simulink model "TorqueVectoring_6_1"  (R2023a)
settings: Solver=FixedStepAuto  StartTime=0.0  StopTime=8  FixedStep=.001  RelTol=1e-3
model workspace (MAT data in the model file):
  slipTarget : Simulink.Parameter (value not decoded)
values from neighbouring files (symbols this model uses):
  Kd_slip = 0    [Main_TorqueVectoring_5_1.m]
  Kd_yaw = 0    [Main_TorqueVectoring_5_1.m]
  Ki_slip = 50    [Main_TorqueVectoring_5_1.m]
  Ki_yaw = 10    [Main_TorqueVectoring_5_1.m]
  Kp_slip = 250    [Main_TorqueVectoring_5_1.m]
  Kp_yaw = 100    [Main_TorqueVectoring_5_1.m]
  slip_windupLower = -inf    [Main_TorqueVectoring_5_1.m]
  slip_windupUpper = inf    [Main_TorqueVectoring_5_1.m]
  slipTarget = .2    (= 0.2)    [Main_TorqueVectoring_5_1.m]
  steering = table2array(yawrateSteering)    [Main_TorqueVectoring_5_1.m]
  yaw_prev_error = 0    [Main_TorqueVectoring_5_1.m]
  yawRate = table2array(yawrateTable)    [Main_TorqueVectoring_5_1.m]
  yawrateVelocity = [0, 5, 10, 15, 20, 25, 30, 35]    [Main_TorqueVectoring_5_1.m]
undefined symbols (not defined in the file or in its folder): sigbuilder_block, VehicleVelocity
libraries: slpidlib x6
(part 3 of 4)

== system TorqueVectoring_6_1/Vehicle Dynamics Model/14 DOF MODEL/Subsys Tire/Subsys tfl2/Subsys Fx ==
  note: B
  note: Bx
  note: Bx - atanBX
  note: X
  note: x
  S : Inport
  Fz : Inport  Port=2
  Bx : Product  RndMeth=Zero
  C : Constant  Value=1.65
  Divide : Product  Inputs=*/
  Gain : Gain  Gain=100
  Product{1..4} (4 alike) : Product  RndMeth=Zero
  Scope2 : Scope
  Sh2 : Constant  Value=0
  Subsys BCD : Subsystem
  Subsys D : Subsystem
  SubsysE : Subsystem
  Subtract : Sum  Inputs=+-
  Subtract1 : Sum  Inputs=+-
  Subtract3 : Sum
  Subtract4 : Sum
  Sv : Constant  Value=0
  To Workspace1 : ToWorkspace  VariableName=Fxrls  SampleTime=-1
  atan : Trigonometry  Operator=atan
  atanBx : Trigonometry  Operator=atan
  atanBx1 : Trigonometry
  Fx : Outport
  wires:
  C/1 -> Product2/1, Product3/2
  Subsys D/1(D) -> Product2/2, Product4/2
  Subsys BCD/1(BCD) -> Divide/1
  Product2/1 -> Divide/2
  Subtract3/1 -> Scope2/1, To Workspace1/1, Fx/1
  Product4/1 -> Subtract3/1
  Product3/1 -> atanBx1/1
  atanBx1/1 -> Product4/1
  atan/1 -> Product3/1
  S/1 -> Gain/1
  Subtract4/1 -> Bx/1
  Sv/1 -> Subtract3/2
  Subtract1/1 -> atan/1
  Product1/1 -> Subtract1/2
  SubsysE/1(E) -> Product1/2
  Subtract/1 -> Product1/1
  atanBx/1 -> Subtract/2
  Bx/1 -> Subtract/1, Subtract1/1, atanBx/1
  Divide/1 -> Bx/2
  Sh2/1 -> Subtract4/2
  Fz/1 -> Subsys BCD/1(Fz), Subsys D/1(Fz), SubsysE/1(Fz)
  Gain/1 -> Subtract4/1

== system TorqueVectoring_6_1/Vehicle Dynamics Model/14 DOF MODEL/Subsys Tire/Subsys tfl2/Subsys Fy ==
  note: B
  note: Bx
  note: Bx - atanBX
  note: X
  note: x
  note: Sh
  alpha : Inport
  Fz : Inport  Port=2
  Bx : Product  RndMeth=Zero
  C : Constant  Value=1.3
  Divide : Product  Inputs=*/
  Product{1..4} (4 alike) : Product  RndMeth=Zero
  Scope2 : Scope
  Subsys BCD : Subsystem
  Subsys D : Subsystem
  SubsysE : Subsystem
  Subtract : Sum  Inputs=+-
  Subtract1 : Sum  Inputs=+-
  Subtract3 : Sum
  Subtract4 : Sum
  Sv : Constant  Value=0
  Sv1 : Constant  Value=0
  To Workspace1 : ToWorkspace  VariableName=Fyrls  SampleTime=-1
  atan : Trigonometry  Operator=atan
  atanBx : Trigonometry  Operator=atan
  atanBx1 : Trigonometry
  Fy : Outport
  wires:
  C/1 -> Product2/1, Product3/2
  Subsys D/1(D) -> Product2/2, Product4/2
  Product2/1 -> Divide/2
  Subtract3/1 -> Scope2/1, To Workspace1/1, Fy/1
  Product4/1 -> Subtract3/1
  Product3/1 -> atanBx1/1
  atanBx1/1 -> Product4/1
  atan/1 -> Product3/1
  Subtract4/1 -> Bx/1
  Sv/1 -> Subtract3/2
  Subtract1/1 -> atan/1
  Product1/1 -> Subtract1/2
  SubsysE/1(E) -> Product1/2
  Subtract/1 -> Product1/1
  atanBx/1 -> Subtract/2
  Bx/1 -> Subtract/1, Subtract1/1, atanBx/1
  Divide/1 -> Bx/2
  Sv1/1 -> Subtract4/2
  Subsys BCD/1(BCD) -> Divide/1
  alpha/1 -> Subtract4/1
  Fz/1 -> Subsys BCD/1(Fz), Subsys D/1(Fz), SubsysE/1(Fz)

== system TorqueVectoring_6_1/Vehicle Dynamics Model/14 DOF MODEL/Subsys Tire/Subsys tfl2/Subsys Mz ==
  note: B
  note: Bx
  note: Bx - atanBX
  note: X
  note: x
  alpha : Inport
  Fz : Inport  Port=2
  Bx : Product  RndMeth=Zero
  C : Constant  Value=2.40
  Divide : Product  Inputs=*/
  Product{1..4} (4 alike) : Product  RndMeth=Zero
  Scope2 : Scope
  Sh2 : Constant  Value=0
  Subsys BCD : Subsystem
  Subsys D : Subsystem
  SubsysE : Subsystem
  Subtract : Sum  Inputs=+-
  Subtract1 : Sum  Inputs=+-
  Subtract3 : Sum
  Subtract4 : Sum
  Sv2 : Constant  Value=0
  To Workspace1 : ToWorkspace  VariableName=Mzrls  SampleTime=-1
  atan : Trigonometry  Operator=atan
  atanBx : Trigonometry  Operator=atan
  atanBx1 : Trigonometry
  Mz : Outport
  wires:
  C/1 -> Product2/1, Product3/2
  Subsys D/1(D) -> Product2/2, Product4/2
  Subsys BCD/1(BCD) -> Divide/1
  Product2/1 -> Divide/2
  Subtract3/1 -> Scope2/1, To Workspace1/1, Mz/1
  Product4/1 -> Subtract3/1
  Product3/1 -> atanBx1/1
  atanBx1/1 -> Product4/1
  atan/1 -> Product3/1
  alpha/1 -> Subtract4/1
  Subtract4/1 -> Bx/1
  Sv2/1 -> Subtract3/2
  Subtract1/1 -> atan/1
  Product1/1 -> Subtract1/2
  SubsysE/1(E) -> Product1/2
  Subtract/1 -> Product1/1
  atanBx/1 -> Subtract/2
  Bx/1 -> Subtract/1, Subtract1/1, atanBx/1
  Divide/1 -> Bx/2
  Sh2/1 -> Subtract4/2
  Fz/1 -> Subsys BCD/1(Fz), Subsys D/1(Fz), SubsysE/1(Fz)

== system TorqueVectoring_6_1/Vehicle Dynamics Model/14 DOF MODEL/Subsys Tire/Subsys tfl3/Subsys Fx ==
  note: x
  note: X
  note: Bx - atanBX
  note: Bx
  note: B
  S : Inport
  Fz : Inport  Port=2
  Bx : Product  RndMeth=Zero
  C : Constant  Value=1.65
  Divide : Product  Inputs=*/
  Gain : Gain  Gain=100
  Product{1..4} (4 alike) : Product  RndMeth=Zero
  Scope2 : Scope
  Sh2 : Constant  Value=0
  Subsys BCD : Subsystem
  Subsys D : Subsystem
  SubsysE : Subsystem
  Subtract : Sum  Inputs=+-
  Subtract1 : Sum  Inputs=+-
  Subtract3 : Sum
  Subtract4 : Sum
  Sv : Constant  Value=0
  To Workspace1 : ToWorkspace  VariableName=Fxrrs  SampleTime=-1
  atan : Trigonometry  Operator=atan
  atanBx : Trigonometry  Operator=atan
  atanBx1 : Trigonometry
  Fx : Outport
  wires:
  Gain/1 -> Subtract4/1
  Fz/1 -> SubsysE/1(Fz), Subsys D/1(Fz), Subsys BCD/1(Fz)
  Sh2/1 -> Subtract4/2
  Divide/1 -> Bx/2
  Bx/1 -> atanBx/1, Subtract1/1, Subtract/1
  atanBx/1 -> Subtract/2
  Subtract/1 -> Product1/1
  SubsysE/1(E) -> Product1/2
  Product1/1 -> Subtract1/2
  Subtract1/1 -> atan/1
  Sv/1 -> Subtract3/2
  Subtract4/1 -> Bx/1
  S/1 -> Gain/1
  atan/1 -> Product3/1
  atanBx1/1 -> Product4/1
  Product3/1 -> atanBx1/1
  Product4/1 -> Subtract3/1
  Subtract3/1 -> To Workspace1/1, Fx/1, Scope2/1
  Product2/1 -> Divide/2
  Subsys BCD/1(BCD) -> Divide/1
  Subsys D/1(D) -> Product4/2, Product2/2
  C/1 -> Product3/2, Product2/1

== system TorqueVectoring_6_1/Vehicle Dynamics Model/14 DOF MODEL/Subsys Tire/Subsys tfl3/Subsys Fy ==
  note: Sh
  note: x
  note: X
  note: Bx - atanBX
  note: Bx
  note: B
  alpha : Inport
  Fz : Inport  Port=2
  Bx : Product  RndMeth=Zero
  C : Constant  Value=1.3
  Divide : Product  Inputs=*/
  Product{1..4} (4 alike) : Product  RndMeth=Zero
  Scope2 : Scope
  Subsys BCD : Subsystem
  Subsys D : Subsystem
  SubsysE : Subsystem
  Subtract : Sum  Inputs=+-
  Subtract1 : Sum  Inputs=+-
  Subtract3 : Sum
  Subtract4 : Sum
  Sv : Constant  Value=0
  Sv1 : Constant  Value=0
  To Workspace1 : ToWorkspace  VariableName=Fyrrs  SampleTime=-1
  atan : Trigonometry  Operator=atan
  atanBx : Trigonometry  Operator=atan
  atanBx1 : Trigonometry
  Fy : Outport
  wires:
  Fz/1 -> SubsysE/1(Fz), Subsys D/1(Fz), Subsys BCD/1(Fz)
  alpha/1 -> Subtract4/1
  Subsys BCD/1(BCD) -> Divide/1
  Sv1/1 -> Subtract4/2
  Divide/1 -> Bx/2
  Bx/1 -> atanBx/1, Subtract1/1, Subtract/1
  atanBx/1 -> Subtract/2
  Subtract/1 -> Product1/1
  SubsysE/1(E) -> Product1/2
  Product1/1 -> Subtract1/2
  Subtract1/1 -> atan/1
  Sv/1 -> Subtract3/2
  Subtract4/1 -> Bx/1
  atan/1 -> Product3/1
  atanBx1/1 -> Product4/1
  Product3/1 -> atanBx1/1
  Product4/1 -> Subtract3/1
  Subtract3/1 -> Fy/1, To Workspace1/1, Scope2/1
  Product2/1 -> Divide/2
  Subsys D/1(D) -> Product4/2, Product2/2
  C/1 -> Product3/2, Product2/1

== system TorqueVectoring_6_1/Vehicle Dynamics Model/14 DOF MODEL/Subsys Tire/Subsys tfl3/Subsys Mz ==
  note: x
  note: X
  note: Bx - atanBX
  note: Bx
  note: B
  alpha : Inport
  Fz : Inport  Port=2
  Bx : Product  RndMeth=Zero
  C : Constant  Value=2.40
  Divide : Product  Inputs=*/
  Product{1..4} (4 alike) : Product  RndMeth=Zero
  Scope2 : Scope
  Sh2 : Constant  Value=0
  Subsys BCD : Subsystem
  Subsys D : Subsystem
  SubsysE : Subsystem
  Subtract : Sum  Inputs=+-
  Subtract1 : Sum  Inputs=+-
  Subtract3 : Sum
  Subtract4 : Sum
  Sv2 : Constant  Value=0
  To Workspace1 : ToWorkspace  VariableName=Mzrrs  SampleTime=-1
  atan : Trigonometry  Operator=atan
  atanBx : Trigonometry  Operator=atan
  atanBx1 : Trigonometry
  Mz : Outport
  wires:
  Fz/1 -> SubsysE/1(Fz), Subsys D/1(Fz), Subsys BCD/1(Fz)
  Sh2/1 -> Subtract4/2
  Divide/1 -> Bx/2
  Bx/1 -> atanBx/1, Subtract1/1, Subtract/1
  atanBx/1 -> Subtract/2
  Subtract/1 -> Product1/1
  SubsysE/1(E) -> Product1/2
  Product1/1 -> Subtract1/2
  Subtract1/1 -> atan/1
  Sv2/1 -> Subtract3/2
  Subtract4/1 -> Bx/1
  alpha/1 -> Subtract4/1
  atan/1 -> Product3/1
  atanBx1/1 -> Product4/1
  Product3/1 -> atanBx1/1
  Product4/1 -> Subtract3/1
  Subtract3/1 -> Mz/1, To Workspace1/1, Scope2/1
  Product2/1 -> Divide/2
  Subsys BCD/1(BCD) -> Divide/1
  Subsys D/1(D) -> Product4/2, Product2/2
  C/1 -> Product3/2, Product2/1

== system TorqueVectoring_6_1/Vehicle Dynamics Model/14 DOF MODEL/Subsys ride/Subsys Fz/Subsys Fzfl ==
  note: mufl.g
  note: Ms.g
  note: Ms.gb
  note: a+b
  note: 2(a+b)
  note: Msg.b/2(a+b)
  Ffl : Inport
  Add : Sum
  Add1 : Sum  Inputs=+++
  Divide : Product  Inputs=*/
  Ms : Constant  Value=Ms
  Product3 : Product  RndMeth=Zero
  a : Constant  Value=a
  b : Constant  Value=b
  constant : Gain  Gain=2
  g : Gain  Gain=9.81
  g1 : Gain  Gain=9.81
  mufl : Constant  Value=mufl
  Fzfl : Outport
  wires:
  b/1 -> Product3/2, Add/1
  Product3/1 -> Divide/1
  a/1 -> Add/2
  Add/1 -> constant/1
  constant/1 -> Divide/2
  mufl/1 -> g/1
  g/1 -> Add1/2
  Ms/1 -> g1/1
  g1/1 -> Product3/1
  Divide/1 -> Add1/1
  Ffl/1 -> Add1/3
  Add1/1 -> Fzfl/1

== system TorqueVectoring_6_1/Vehicle Dynamics Model/14 DOF MODEL/Subsys ride/Subsys Fz/Subsys Fzfr ==
  note: Msg.b/2(a+b)
  note: 2(a+b)
  note: a+b
  note: Ms.gb
  note: Ms.g
  note: mufr.g
  Ffr : Inport
  Add : Sum
  Add1 : Sum  Inputs=+++
  Divide : Product  Inputs=*/
  Ms : Constant  Value=Ms
  Product3 : Product  RndMeth=Zero
  a : Constant  Value=a
  b : Constant  Value=b
  constant : Gain  Gain=2
  g : Gain  Gain=9.81
  g1 : Gain  Gain=9.81
  mufr : Constant  Value=mufr
  Fzfr : Outport
  wires:
  Add1/1 -> Fzfr/1
  Ffr/1 -> Add1/3
  Divide/1 -> Add1/1
  g1/1 -> Product3/1
  Ms/1 -> g1/1
  g/1 -> Add1/2
  mufr/1 -> g/1
  constant/1 -> Divide/2
  Add/1 -> constant/1
  a/1 -> Add/2
  Product3/1 -> Divide/1
  b/1 -> Add/1, Product3/2

== system TorqueVectoring_6_1/Vehicle Dynamics Model/14 DOF MODEL/Subsys ride/Subsys Fz/Subsys Fzrl ==
  note: Msg.a/2(a+b)
  note: 2(a+b)
  note: a+b
  note: Ms.ga
  note: Ms.g
  note: murl.g
  Frl : Inport
  Add : Sum
  Add1 : Sum  Inputs=+++
  Divide : Product  Inputs=*/
  Ms : Constant  Value=Ms
  Product3 : Product  RndMeth=Zero
  a : Constant  Value=a
  b : Constant  Value=b
  constant : Gain  Gain=2
  g : Gain  Gain=9.81
  g1 : Gain  Gain=9.81
  mufl : Constant  Value=murl
  Fzrl : Outport
  wires:
  Add1/1 -> Fzrl/1
  Frl/1 -> Add1/3
  Divide/1 -> Add1/1
  g1/1 -> Product3/1
  Ms/1 -> g1/1
  g/1 -> Add1/2
  mufl/1 -> g/1
  constant/1 -> Divide/2
  Add/1 -> constant/1
  b/1 -> Add/2
  Product3/1 -> Divide/1
  a/1 -> Add/1, Product3/2

== system TorqueVectoring_6_1/Vehicle Dynamics Model/14 DOF MODEL/Subsys ride/Subsys Fz/Subsys Fzrl1 ==
  note: murr.g
  note: Ms.g
  note: Ms.ga
  note: a+b
  note: 2(a+b)
  note: Msg.a/2(a+b)
  Frr : Inport
  Add : Sum
  Add1 : Sum  Inputs=+++
  Divide : Product  Inputs=*/
  Ms : Constant  Value=Ms
  Product3 : Product  RndMeth=Zero
  a : Constant  Value=a
  b : Constant  Value=b
  constant : Gain  Gain=2
  g : Gain  Gain=9.81
  g1 : Gain  Gain=9.81
  murr : Constant  Value=murr
  Fzrr : Outport
  wires:
  a/1 -> Product3/2, Add/1
  Product3/1 -> Divide/1
  b/1 -> Add/2
  Add/1 -> constant/1
  constant/1 -> Divide/2
  murr/1 -> g/1
  g/1 -> Add1/2
  Ms/1 -> g1/1
  g1/1 -> Product3/1
  Divide/1 -> Add1/1
  Frr/1 -> Add1/3
  Add1/1 -> Fzrr/1

== system TorqueVectoring_6_1/Vehicle Dynamics Model/14 DOF MODEL/Subsys ride/Subsys wheel fl/Ftfl ==
  Zrfl : Inport
  Zufl : Inport  Port=2
  Gain : Gain  Gain=Ktfl
  Subtract : Sum  Inputs=+-
  Ftfl : Outport
  wires:
  Subtract/1 -> Gain/1
  Zrfl/1 -> Subtract/1
  Zufl/1 -> Subtract/2
  Gain/1 -> Ftfl/1

== system TorqueVectoring_6_1/Vehicle Dynamics Model/14 DOF MODEL/Subsys ride/Subsys wheel fr/Ftfr ==
  Zrfr : Inport
  Zufr : Inport  Port=2
  Gain : Gain  Gain=Ktfr
  Subtract : Sum  Inputs=+-
  Ftfr : Outport
  wires:
  Gain/1 -> Ftfr/1
  Zufr/1 -> Subtract/2
  Zrfr/1 -> Subtract/1
  Subtract/1 -> Gain/1

== system TorqueVectoring_6_1/Vehicle Dynamics Model/14 DOF MODEL/Subsys ride/Subsys wheel rl/Ftrl ==
  Zrrl : Inport
  Zurl : Inport  Port=2
  Gain : Gain  Gain=Ktrl
  Subtract : Sum  Inputs=+-
  Ftrl : Outport
  wires:
  Subtract/1 -> Gain/1
  Zrrl/1 -> Subtract/1
  Zurl/1 -> Subtract/2
  Gain/1 -> Ftrl/1

== system TorqueVectoring_6_1/Vehicle Dynamics Model/14 DOF MODEL/Subsys ride/Subsys wheel rr/Ftfr2 ==
  Zrrr : Inport
  Zurr : Inport  Port=2
  Gain : Gain  Gain=Ktrr
  Subtract : Sum  Inputs=+-
  Ftfr : Outport
  wires:
  Gain/1 -> Ftfr/1
  Zurr/1 -> Subtract/2
  Zrrr/1 -> Subtract/1
  Subtract/1 -> Gain/1

== system TorqueVectoring_6_1/Vehicle Dynamics Model/14 DOF MODEL/Subsys Tire/Subsys tfl/Subsys Fx/Subsys BCD (Cornering Stiffness) ==
  Fz : Inport
  Add : Sum
  Divide : Product  Inputs=*/
  Fz^1 : Math  SignedPower=on
  Fz^2 : Math  Operator=square  SignedPower=on
  Product1 : Product  RndMeth=Zero
  Product2 : Product  RndMeth=Zero
  Product3 : Product  RndMeth=Zero
  a3 : Constant  Value=49.6
  a4 : Constant  Value=226
  a5 : Constant  Value=0.069
  BCD : Outport
  wires:
  Fz/1 -> Fz^2/1, Product1/2, Product3/2
  a4/1 -> Product1/1
  a3/1 -> Product2/1
  Fz^2/1 -> Product2/2
  Product2/1 -> Add/1
  Product1/1 -> Add/2
  a5/1 -> Product3/1
  Product3/1 -> Fz^1/1
  Add/1 -> Divide/1
  Fz^1/1 -> Divide/2
  Divide/1 -> BCD/1

== system TorqueVectoring_6_1/Vehicle Dynamics Model/14 DOF MODEL/Subsys Tire/Subsys tfl/Subsys Fx/Subsys D ==
  Fz : Inport
  Add1 : Sum
  Fz^2 : Math  Operator=square  SignedPower=on
  Product : Product  RndMeth=Zero
  Product1 : Product  RndMeth=Zero
  a1 : Constant  Value=-21.3
  a2 : Constant  Value=1144
  D : Outport
  wires:
  Fz/1 -> Fz^2/1, Product1/2
  a1/1 -> Product/1
  Fz^2/1 -> Product/2
  a2/1 -> Product1/1
  Product1/1 -> Add1/2
  Product/1 -> Add1/1
  Add1/1 -> D/1

== system TorqueVectoring_6_1/Vehicle Dynamics Model/14 DOF MODEL/Subsys Tire/Subsys tfl/Subsys Fx/SubsysE ==
  Fz : Inport
  Add : Sum  Inputs=+++
  Fz^2 : Math  Operator=square  SignedPower=on
  Product1 : Product  RndMeth=Zero
  Product3 : Product  RndMeth=Zero
  a6 : Constant  Value=-0.006
  a7 : Constant  Value=0.056
  a8 : Constant  Value=0.486
  E : Outport
  wires:
  Fz/1 -> Fz^2/1, Product1/2
  a7/1 -> Product1/1
  a6/1 -> Product3/1
  Fz^2/1 -> Product3/2
  Product3/1 -> Add/1
  Product1/1 -> Add/2
  Add/1 -> E/1
  a8/1 -> Add/3

== system TorqueVectoring_6_1/Vehicle Dynamics Model/14 DOF MODEL/Subsys Tire/Subsys tfl/Subsys Fy/Subsys BCD ==
  Fz : Inport
  Product1 : Product  RndMeth=Zero
  Product2 : Product  RndMeth=Zero
  Product3 : Product  RndMeth=Zero
  Trigonometric Function : Trigonometry  Operator=atan
  Trigonometric Function1 : Trigonometry
  a3 : Constant  Value=1078
  a4 : Constant  Value=1.82
  a5 : Constant  Value=0.208
  BCD : Outport
  wires:
  Fz/1 -> Product2/2
  a5/1 -> Product2/1
  Product2/1 -> Trigonometric Function/1
  Trigonometric Function/1 -> Product1/2
  a4/1 -> Product1/1
  Product1/1 -> Trigonometric Function1/1
  Trigonometric Function1/1 -> Product3/2
  a3/1 -> Product3/1
  Product3/1 -> BCD/1

== system TorqueVectoring_6_1/Vehicle Dynamics Model/14 DOF MODEL/Subsys Tire/Subsys tfl/Subsys Fy/Subsys D ==
  Fz : Inport
  Add1 : Sum
  Fz^2 : Math  Operator=square  SignedPower=on
  Product : Product  RndMeth=Zero
  Product1 : Product  RndMeth=Zero
  a1 : Constant  Value=-22.1
  a2 : Constant  Value=1011
  D : Outport
  wires:
  Fz/1 -> Fz^2/1, Product1/2
  a1/1 -> Product/1
  Fz^2/1 -> Product/2
  a2/1 -> Product1/1
  Product1/1 -> Add1/2
  Product/1 -> Add1/1
  Add1/1 -> D/1

== system TorqueVectoring_6_1/Vehicle Dynamics Model/14 DOF MODEL/Subsys Tire/Subsys tfl/Subsys Fy/SubsysE ==
  Fz : Inport
  Add : Sum  Inputs=+++
  Fz^2 : Math  Operator=square  SignedPower=on
  Product1 : Product  RndMeth=Zero
  Product3 : Product  RndMeth=Zero
  a6 : Constant  Value=0.0000
  a7 : Constant  Value=-0.354
  a8 : Constant  Value=0.707
  E : Outport
  wires:
  Fz/1 -> Fz^2/1, Product1/2
  a7/1 -> Product1/1
  a6/1 -> Product3/1
  Fz^2/1 -> Product3/2
  Product3/1 -> Add/1
  Product1/1 -> Add/2
  Add/1 -> E/1
  a8/1 -> Add/3

== system TorqueVectoring_6_1/Vehicle Dynamics Model/14 DOF MODEL/Subsys Tire/Subsys tfl/Subsys Mz/Subsys BCD ==
  Fz : Inport
  Add : Sum
  Divide : Product  Inputs=*/
  Fz^1 : Math  SignedPower=on
  Fz^2 : Math  Operator=square  SignedPower=on
  Product1 : Product  RndMeth=Zero
  Product2 : Product  RndMeth=Zero
  Product3 : Product  RndMeth=Zero
  a3 : Constant  Value=-1.86
  a4 : Constant  Value=-2.73
  a5 : Constant  Value=0.110
  BCD : Outport
  wires:
  Fz/1 -> Fz^2/1, Product1/2, Product3/2
  a4/1 -> Product1/1
  a3/1 -> Product2/1
  Fz^2/1 -> Product2/2
  Product2/1 -> Add/1
  Product1/1 -> Add/2
  a5/1 -> Product3/1
  Product3/1 -> Fz^1/1
  Add/1 -> Divide/1
  Fz^1/1 -> Divide/2
  Divide/1 -> BCD/1

== system TorqueVectoring_6_1/Vehicle Dynamics Model/14 DOF MODEL/Subsys Tire/Subsys tfl/Subsys Mz/Subsys D ==
  Fz : Inport
  Add1 : Sum
  Fz^2 : Math  Operator=square  SignedPower=on
  Product : Product  RndMeth=Zero
  Product1 : Product  RndMeth=Zero
  a1 : Constant  Value=-2.72
  a2 : Constant  Value=-2.28
  D : Outport
  wires:
  Fz/1 -> Fz^2/1, Product1/2
  a1/1 -> Product/1
  Fz^2/1 -> Product/2
  a2/1 -> Product1/1
  Product1/1 -> Add1/2
  Product/1 -> Add1/1
  Add1/1 -> D/1

== system TorqueVectoring_6_1/Vehicle Dynamics Model/14 DOF MODEL/Subsys Tire/Subsys tfl/Subsys Mz/SubsysE ==
  Fz : Inport
  Add : Sum  Inputs=+++
  Fz^2 : Math  Operator=square  SignedPower=on
  Product1 : Product  RndMeth=Zero
  Product3 : Product  RndMeth=Zero
  a6 : Constant  Value=-0.070
  a7 : Constant  Value=0.643
  a8 : Constant  Value=-4.04
  E : Outport
  wires:
  Fz/1 -> Fz^2/1, Product1/2
  a7/1 -> Product1/1
  a6/1 -> Product3/1
  Fz^2/1 -> Product3/2
  Product3/1 -> Add/1
  Product1/1 -> Add/2
  Add/1 -> E/1
  a8/1 -> Add/3

== system TorqueVectoring_6_1/Vehicle Dynamics Model/14 DOF MODEL/Subsys Tire/Subsys tfl1/Subsys Fx/Subsys BCD ==
  Fz : Inport
  Add : Sum
  Divide : Product  Inputs=*/
  Fz^1 : Math  SignedPower=on
  Fz^2 : Math  Operator=square  SignedPower=on
  Product1 : Product  RndMeth=Zero
  Product2 : Product  RndMeth=Zero
  Product3 : Product  RndMeth=Zero
  a3 : Constant  Value=49.6
  a4 : Constant  Value=226
  a5 : Constant  Value=0.069
  BCD : Outport
  wires:
  Divide/1 -> BCD/1
  Fz^1/1 -> Divide/2
  Add/1 -> Divide/1
  Product3/1 -> Fz^1/1
  a5/1 -> Product3/1
  Product1/1 -> Add/2
  Product2/1 -> Add/1
  Fz^2/1 -> Product2/2
  a3/1 -> Product2/1
  a4/1 -> Product1/1
  Fz/1 -> Product3/2, Product1/2, Fz^2/1

== system TorqueVectoring_6_1/Vehicle Dynamics Model/14 DOF MODEL/Subsys Tire/Subsys tfl1/Subsys Fx/Subsys D ==
  Fz : Inport
  Add1 : Sum
  Fz^2 : Math  Operator=square  SignedPower=on
  Product : Product  RndMeth=Zero
  Product1 : Product  RndMeth=Zero
  a1 : Constant  Value=-21.3
  a2 : Constant  Value=1144
  D : Outport
  wires:
  Add1/1 -> D/1
  Product/1 -> Add1/1
  Product1/1 -> Add1/2
  a2/1 -> Product1/1
  Fz^2/1 -> Product/2
  a1/1 -> Product/1
  Fz/1 -> Product1/2, Fz^2/1

== system TorqueVectoring_6_1/Vehicle Dynamics Model/14 DOF MODEL/Subsys Tire/Subsys tfl1/Subsys Fx/SubsysE ==
  Fz : Inport
  Add : Sum  Inputs=+++
  Fz^2 : Math  Operator=square  SignedPower=on
  Product1 : Product  RndMeth=Zero
  Product3 : Product  RndMeth=Zero
  a6 : Constant  Value=-0.006
  a7 : Constant  Value=0.056
  a8 : Constant  Value=0.486
  E : Outport
  wires:
  a8/1 -> Add/3
  Add/1 -> E/1
  Product1/1 -> Add/2
  Product3/1 -> Add/1
  Fz^2/1 -> Product3/2
  a6/1 -> Product3/1
  a7/1 -> Product1/1
  Fz/1 -> Product1/2, Fz^2/1

== system TorqueVectoring_6_1/Vehicle Dynamics Model/14 DOF MODEL/Subsys Tire/Subsys tfl1/Subsys Fy/Subsys BCD ==
  Fz : Inport
  Product1 : Product  RndMeth=Zero
  Product2 : Product  RndMeth=Zero
  Product3 : Product  RndMeth=Zero
  Trigonometric Function : Trigonometry  Operator=atan
  Trigonometric Function1 : Trigonometry
  a3 : Constant  Value=1078
  a4 : Constant  Value=1.82
  a5 : Constant  Value=0.208
  BCD : Outport
  wires:
  Product3/1 -> BCD/1
  a3/1 -> Product3/1
  Trigonometric Function1/1 -> Product3/2
  Product1/1 -> Trigonometric Function1/1
  a4/1 -> Product1/1
  Trigonometric Function/1 -> Product1/2
  Product2/1 -> Trigonometric Function/1
  a5/1 -> Product2/1
  Fz/1 -> Product2/2

== system TorqueVectoring_6_1/Vehicle Dynamics Model/14 DOF MODEL/Subsys Tire/Subsys tfl1/Subsys Fy/Subsys D ==
  Fz : Inport
  Add1 : Sum
  Fz^2 : Math  Operator=square  SignedPower=on
  Product : Product  RndMeth=Zero
  Product1 : Product  RndMeth=Zero
  a1 : Constant  Value=-22.1
  a2 : Constant  Value=1011
  D : Outport
  wires:
  Add1/1 -> D/1
  Product/1 -> Add1/1
  Product1/1 -> Add1/2
  a2/1 -> Product1/1
  Fz^2/1 -> Product/2
  a1/1 -> Product/1
  Fz/1 -> Product1/2, Fz^2/1

== system TorqueVectoring_6_1/Vehicle Dynamics Model/14 DOF MODEL/Subsys Tire/Subsys tfl1/Subsys Fy/SubsysE ==
  Fz : Inport
  Add : Sum  Inputs=+++
  Fz^2 : Math  Operator=square  SignedPower=on
  Product1 : Product  RndMeth=Zero
  Product3 : Product  RndMeth=Zero
  a6 : Constant  Value=0.0000
  a7 : Constant  Value=-0.354
  a8 : Constant  Value=0.707
  E : Outport
  wires:
  a8/1 -> Add/3
  Add/1 -> E/1
  Product1/1 -> Add/2
  Product3/1 -> Add/1
  Fz^2/1 -> Product3/2
  a6/1 -> Product3/1
  a7/1 -> Product1/1
  Fz/1 -> Product1/2, Fz^2/1

== system TorqueVectoring_6_1/Vehicle Dynamics Model/14 DOF MODEL/Subsys Tire/Subsys tfl1/Subsys Mz/Subsys BCD ==
  Fz : Inport
  Add : Sum
  Divide : Product  Inputs=*/
  Fz^1 : Math  SignedPower=on
  Fz^2 : Math  Operator=square  SignedPower=on
  Product1 : Product  RndMeth=Zero
  Product2 : Product  RndMeth=Zero
  Product3 : Product  RndMeth=Zero
  a3 : Constant  Value=-1.86
  a4 : Constant  Value=-2.73
  a5 : Constant  Value=0.110
  BCD : Outport
  wires:
  Divide/1 -> BCD/1
  Fz^1/1 -> Divide/2
  Add/1 -> Divide/1
  Product3/1 -> Fz^1/1
  a5/1 -> Product3/1
  Product1/1 -> Add/2
  Product2/1 -> Add/1
  Fz^2/1 -> Product2/2
  a3/1 -> Product2/1
  a4/1 -> Product1/1
  Fz/1 -> Product3/2, Product1/2, Fz^2/1

== system TorqueVectoring_6_1/Vehicle Dynamics Model/14 DOF MODEL/Subsys Tire/Subsys tfl1/Subsys Mz/Subsys D ==
  Fz : Inport
  Add1 : Sum
  Fz^2 : Math  Operator=square  SignedPower=on
  Product : Product  RndMeth=Zero
  Product1 : Product  RndMeth=Zero
  a1 : Constant  Value=-2.72
  a2 : Constant  Value=-2.28
  D : Outport
  wires:
  Add1/1 -> D/1
  Product/1 -> Add1/1
  Product1/1 -> Add1/2
  a2/1 -> Product1/1
  Fz^2/1 -> Product/2
  a1/1 -> Product/1
  Fz/1 -> Product1/2, Fz^2/1

== system TorqueVectoring_6_1/Vehicle Dynamics Model/14 DOF MODEL/Subsys Tire/Subsys tfl1/Subsys Mz/SubsysE ==
  Fz : Inport
  Add : Sum  Inputs=+++
  Fz^2 : Math  Operator=square  SignedPower=on
  Product1 : Product  RndMeth=Zero
  Product3 : Product  RndMeth=Zero
  a6 : Constant  Value=-0.070
  a7 : Constant  Value=0.643
  a8 : Constant  Value=-4.04
  E : Outport
  wires:
  a8/1 -> Add/3
  Add/1 -> E/1
  Product1/1 -> Add/2
  Product3/1 -> Add/1
  Fz^2/1 -> Product3/2
  a6/1 -> Product3/1
  a7/1 -> Product1/1
  Fz/1 -> Product1/2, Fz^2/1

== system TorqueVectoring_6_1/Vehicle Dynamics Model/14 DOF MODEL/Subsys Tire/Subsys tfl2/Subsys Fx/Subsys BCD ==
  Fz : Inport
  Add : Sum
  Divide : Product  Inputs=*/
  Fz^1 : Math  SignedPower=on
  Fz^2 : Math  Operator=square  SignedPower=on
  Product1 : Product  RndMeth=Zero
  Product2 : Product  RndMeth=Zero
  Product3 : Product  RndMeth=Zero
  a3 : Constant  Value=49.6
  a4 : Constant  Value=226
  a5 : Constant  Value=0.069
  BCD : Outport
  wires:
  Fz/1 -> Fz^2/1, Product1/2, Product3/2
  a4/1 -> Product1/1
  a3/1 -> Product2/1
  Fz^2/1 -> Product2/2
  Product2/1 -> Add/1
  Product1/1 -> Add/2
  a5/1 -> Product3/1
  Product3/1 -> Fz^1/1
  Add/1 -> Divide/1
  Fz^1/1 -> Divide/2
  Divide/1 -> BCD/1

== system TorqueVectoring_6_1/Vehicle Dynamics Model/14 DOF MODEL/Subsys Tire/Subsys tfl2/Subsys Fx/Subsys D ==
  Fz : Inport
  Add1 : Sum
  Fz^2 : Math  Operator=square  SignedPower=on
  Product : Product  RndMeth=Zero
  Product1 : Product  RndMeth=Zero
  a1 : Constant  Value=-21.3
  a2 : Constant  Value=1144
  D : Outport
  wires:
  Fz/1 -> Fz^2/1, Product1/2
  a1/1 -> Product/1
  Fz^2/1 -> Product/2
  a2/1 -> Product1/1
  Product1/1 -> Add1/2
  Product/1 -> Add1/1
  Add1/1 -> D/1

== system TorqueVectoring_6_1/Vehicle Dynamics Model/14 DOF MODEL/Subsys Tire/Subsys tfl2/Subsys Fx/SubsysE ==
  Fz : Inport
  Add : Sum  Inputs=+++
  Fz^2 : Math  Operator=square  SignedPower=on
  Product1 : Product  RndMeth=Zero
  Product3 : Product  RndMeth=Zero
  a6 : Constant  Value=-0.006
  a7 : Constant  Value=0.056
  a8 : Constant  Value=0.486
  E : Outport
  wires:
  Fz/1 -> Fz^2/1, Product1/2
  a7/1 -> Product1/1
  a6/1 -> Product3/1
  Fz^2/1 -> Product3/2
  Product3/1 -> Add/1
  Product1/1 -> Add/2
  Add/1 -> E/1
  a8/1 -> Add/3

== system TorqueVectoring_6_1/Vehicle Dynamics Model/14 DOF MODEL/Subsys Tire/Subsys tfl2/Subsys Fy/Subsys BCD ==
  Fz : Inport
  Product1 : Product  RndMeth=Zero
  Product2 : Product  RndMeth=Zero
  Product3 : Product  RndMeth=Zero
  Trigonometric Function : Trigonometry  Operator=atan
  Trigonometric Function1 : Trigonometry
  a3 : Constant  Value=1078
  a4 : Constant  Value=1.82
  a5 : Constant  Value=0.208
  BCD : Outport
  wires:
  Fz/1 -> Product2/2
  a5/1 -> Product2/1
  Product2/1 -> Trigonometric Function/1
  Trigonometric Function/1 -> Product1/2
  a4/1 -> Product1/1
  Product1/1 -> Trigonometric Function1/1
  Trigonometric Function1/1 -> Product3/2
  a3/1 -> Product3/1
  Product3/1 -> BCD/1

== system TorqueVectoring_6_1/Vehicle Dynamics Model/14 DOF MODEL/Subsys Tire/Subsys tfl2/Subsys Fy/Subsys D ==
  Fz : Inport
  Add1 : Sum
  Fz^2 : Math  Operator=square  SignedPower=on
  Product : Product  RndMeth=Zero
  Product1 : Product  RndMeth=Zero
  a1 : Constant  Value=-22.1
  a2 : Constant  Value=1011
  D : Outport
  wires:
  Fz/1 -> Fz^2/1, Product1/2
  a1/1 -> Product/1
  Fz^2/1 -> Product/2
  a2/1 -> Product1/1
  Product1/1 -> Add1/2
  Product/1 -> Add1/1
  Add1/1 -> D/1

== system TorqueVectoring_6_1/Vehicle Dynamics Model/14 DOF MODEL/Subsys Tire/Subsys tfl2/Subsys Fy/SubsysE ==
  Fz : Inport
  Add : Sum  Inputs=+++
  Fz^2 : Math  Operator=square  SignedPower=on
  Product1 : Product  RndMeth=Zero
  Product3 : Product  RndMeth=Zero
  a6 : Constant  Value=0.0000
  a7 : Constant  Value=-0.354
  a8 : Constant  Value=0.707
  E : Outport
  wires:
  Fz/1 -> Fz^2/1, Product1/2
  a7/1 -> Product1/1
  a6/1 -> Product3/1
  Fz^2/1 -> Product3/2
  Product3/1 -> Add/1
  Product1/1 -> Add/2
  Add/1 -> E/1
  a8/1 -> Add/3

== system TorqueVectoring_6_1/Vehicle Dynamics Model/14 DOF MODEL/Subsys Tire/Subsys tfl2/Subsys Mz/Subsys BCD ==
  Fz : Inport
  Add : Sum
  Divide : Product  Inputs=*/
  Fz^1 : Math  SignedPower=on
  Fz^2 : Math  Operator=square  SignedPower=on
  Product1 : Product  RndMeth=Zero
  Product2 : Product  RndMeth=Zero
  Product3 : Product  RndMeth=Zero
  a3 : Constant  Value=-1.86
  a4 : Constant  Value=-2.73
  a5 : Constant  Value=0.110
  BCD : Outport
  wires:
  Fz/1 -> Fz^2/1, Product1/2, Product3/2
  a4/1 -> Product1/1
  a3/1 -> Product2/1
  Fz^2/1 -> Product2/2
  Product2/1 -> Add/1
  Product1/1 -> Add/2
  a5/1 -> Product3/1
  Product3/1 -> Fz^1/1
  Add/1 -> Divide/1
  Fz^1/1 -> Divide/2
  Divide/1 -> BCD/1

== system TorqueVectoring_6_1/Vehicle Dynamics Model/14 DOF MODEL/Subsys Tire/Subsys tfl2/Subsys Mz/Subsys D ==
  Fz : Inport
  Add1 : Sum
  Fz^2 : Math  Operator=square  SignedPower=on
  Product : Product  RndMeth=Zero
  Product1 : Product  RndMeth=Zero
  a1 : Constant  Value=-2.72
  a2 : Constant  Value=-2.28
  D : Outport
  wires:
  Fz/1 -> Fz^2/1, Product1/2
  a1/1 -> Product/1
  Fz^2/1 -> Product/2
  a2/1 -> Product1/1
  Product1/1 -> Add1/2
  Product/1 -> Add1/1
  Add1/1 -> D/1

== system TorqueVectoring_6_1/Vehicle Dynamics Model/14 DOF MODEL/Subsys Tire/Subsys tfl2/Subsys Mz/SubsysE ==
  Fz : Inport
  Add : Sum  Inputs=+++
  Fz^2 : Math  Operator=square  SignedPower=on
  Product1 : Product  RndMeth=Zero
  Product3 : Product  RndMeth=Zero
  a6 : Constant  Value=-0.070
  a7 : Constant  Value=0.643
  a8 : Constant  Value=-4.04
  E : Outport
  wires:
  Fz/1 -> Fz^2/1, Product1/2
  a7/1 -> Product1/1
  a6/1 -> Product3/1
  Fz^2/1 -> Product3/2
  Product3/1 -> Add/1
  Product1/1 -> Add/2
  Add/1 -> E/1
  a8/1 -> Add/3

== system TorqueVectoring_6_1/Vehicle Dynamics Model/14 DOF MODEL/Subsys Tire/Subsys tfl3/Subsys Fx/Subsys BCD ==
  Fz : Inport
  Add : Sum
  Divide : Product  Inputs=*/
  Fz^1 : Math  SignedPower=on
  Fz^2 : Math  Operator=square  SignedPower=on
  Product1 : Product  RndMeth=Zero
  Product2 : Product  RndMeth=Zero
  Product3 : Product  RndMeth=Zero
  a3 : Constant  Value=49.6
  a4 : Constant  Value=226
  a5 : Constant  Value=0.069
  BCD : Outport
  wires:
  Divide/1 -> BCD/1
  Fz^1/1 -> Divide/2
  Add/1 -> Divide/1
  Product3/1 -> Fz^1/1
  a5/1 -> Product3/1
  Product1/1 -> Add/2
  Product2/1 -> Add/1
  Fz^2/1 -> Product2/2
  a3/1 -> Product2/1
  a4/1 -> Product1/1
  Fz/1 -> Product3/2, Product1/2, Fz^2/1

== system TorqueVectoring_6_1/Vehicle Dynamics Model/14 DOF MODEL/Subsys Tire/Subsys tfl3/Subsys Fx/Subsys D ==
  Fz : Inport
  Add1 : Sum
  Fz^2 : Math  Operator=square  SignedPower=on
  Product : Product  RndMeth=Zero
  Product1 : Product  RndMeth=Zero
  a1 : Constant  Value=-21.3
  a2 : Constant  Value=1144
  D : Outport
  wires:
  Add1/1 -> D/1
  Product/1 -> Add1/1
  Product1/1 -> Add1/2
  a2/1 -> Product1/1
  Fz^2/1 -> Product/2
  a1/1 -> Product/1
  Fz/1 -> Product1/2, Fz^2/1

== system TorqueVectoring_6_1/Vehicle Dynamics Model/14 DOF MODEL/Subsys Tire/Subsys tfl3/Subsys Fx/SubsysE ==
  Fz : Inport
  Add : Sum  Inputs=+++
  Fz^2 : Math  Operator=square  SignedPower=on
  Product1 : Product  RndMeth=Zero
  Product3 : Product  RndMeth=Zero
  a6 : Constant  Value=-0.006
  a7 : Constant  Value=0.056
  a8 : Constant  Value=0.486
  E : Outport
  wires:
  a8/1 -> Add/3
  Add/1 -> E/1
  Product1/1 -> Add/2
  Product3/1 -> Add/1
  Fz^2/1 -> Product3/2
  a6/1 -> Product3/1
  a7/1 -> Product1/1
  Fz/1 -> Product1/2, Fz^2/1

== system TorqueVectoring_6_1/Vehicle Dynamics Model/14 DOF MODEL/Subsys Tire/Subsys tfl3/Subsys Fy/Subsys BCD ==
  Fz : Inport
  Product1 : Product  RndMeth=Zero
  Product2 : Product  RndMeth=Zero
  Product3 : Product  RndMeth=Zero
  Trigonometric Function : Trigonometry  Operator=atan
  Trigonometric Function1 : Trigonometry
  a3 : Constant  Value=1078
  a4 : Constant  Value=1.82
  a5 : Constant  Value=0.208
  BCD : Outport
  wires:
  Product3/1 -> BCD/1
  a3/1 -> Product3/1
  Trigonometric Function1/1 -> Product3/2
  Product1/1 -> Trigonometric Function1/1
  a4/1 -> Product1/1
  Trigonometric Function/1 -> Product1/2
  Product2/1 -> Trigonometric Function/1
  a5/1 -> Product2/1
  Fz/1 -> Product2/2

== system TorqueVectoring_6_1/Vehicle Dynamics Model/14 DOF MODEL/Subsys Tire/Subsys tfl3/Subsys Fy/Subsys D ==
  Fz : Inport
  Add1 : Sum
  Fz^2 : Math  Operator=square  SignedPower=on
  Product : Product  RndMeth=Zero
  Product1 : Product  RndMeth=Zero
  a1 : Constant  Value=-22.1
  a2 : Constant  Value=1011
  D : Outport
  wires:
  Add1/1 -> D/1
  Product/1 -> Add1/1
  Product1/1 -> Add1/2
  a2/1 -> Product1/1
  Fz^2/1 -> Product/2
  a1/1 -> Product/1
  Fz/1 -> Product1/2, Fz^2/1

== system TorqueVectoring_6_1/Vehicle Dynamics Model/14 DOF MODEL/Subsys Tire/Subsys tfl3/Subsys Fy/SubsysE ==
  Fz : Inport
  Add : Sum  Inputs=+++
  Fz^2 : Math  Operator=square  SignedPower=on
  Product1 : Product  RndMeth=Zero
  Product3 : Product  RndMeth=Zero
  a6 : Constant  Value=0.0000
  a7 : Constant  Value=-0.354
  a8 : Constant  Value=0.707
  E : Outport
  wires:
  a8/1 -> Add/3
  Add/1 -> E/1
  Product1/1 -> Add/2
  Product3/1 -> Add/1
  Fz^2/1 -> Product3/2
  a6/1 -> Product3/1
  a7/1 -> Product1/1
  Fz/1 -> Product1/2, Fz^2/1

== system TorqueVectoring_6_1/Vehicle Dynamics Model/14 DOF MODEL/Subsys Tire/Subsys tfl3/Subsys Mz/Subsys BCD ==
  Fz : Inport
  Add : Sum
  Divide : Product  Inputs=*/
  Fz^1 : Math  SignedPower=on
  Fz^2 : Math  Operator=square  SignedPower=on
  Product1 : Product  RndMeth=Zero
  Product2 : Product  RndMeth=Zero
  Product3 : Product  RndMeth=Zero
  a3 : Constant  Value=-1.86
  a4 : Constant  Value=-2.73
  a5 : Constant  Value=0.110
  BCD : Outport
  wires:
  Divide/1 -> BCD/1
  Fz^1/1 -> Divide/2
  Add/1 -> Divide/1
  Product3/1 -> Fz^1/1
  a5/1 -> Product3/1
  Product1/1 -> Add/2
  Product2/1 -> Add/1
  Fz^2/1 -> Product2/2
  a3/1 -> Product2/1
  a4/1 -> Product1/1
  Fz/1 -> Product3/2, Product1/2, Fz^2/1

== system TorqueVectoring_6_1/Vehicle Dynamics Model/14 DOF MODEL/Subsys Tire/Subsys tfl3/Subsys Mz/Subsys D ==
  Fz : Inport
  Add1 : Sum
  Fz^2 : Math  Operator=square  SignedPower=on
  Product : Product  RndMeth=Zero
  Product1 : Product  RndMeth=Zero
  a1 : Constant  Value=-2.72
  a2 : Constant  Value=-2.28
  D : Outport
  wires:
  Add1/1 -> D/1
  Product/1 -> Add1/1
  Product1/1 -> Add1/2
  a2/1 -> Product1/1
  Fz^2/1 -> Product/2
  a1/1 -> Product/1
  Fz/1 -> Product1/2, Fz^2/1

== system TorqueVectoring_6_1/Vehicle Dynamics Model/14 DOF MODEL/Subsys Tire/Subsys tfl3/Subsys Mz/SubsysE ==
  Fz : Inport
  Add : Sum  Inputs=+++
  Fz^2 : Math  Operator=square  SignedPower=on
  Product1 : Product  RndMeth=Zero
  Product3 : Product  RndMeth=Zero
  a6 : Constant  Value=-0.070
  a7 : Constant  Value=0.643
  a8 : Constant  Value=-4.04
  E : Outport
  wires:
  a8/1 -> Add/3
  Add/1 -> E/1
  Product1/1 -> Add/2
  Product3/1 -> Add/1
  Fz^2/1 -> Product3/2
  a6/1 -> Product3/1
  a7/1 -> Product1/1
  Fz/1 -> Product1/2, Fz^2/1

== matlab function TorqueVectoring_6_1/Traction Control/RL/MATLAB Function ==
  data: enable output; actualSlip input; setpoint output; SlipTarget input
function [enable,setpoint] = slipCtrlTrigger(actualSlip,SlipTarget)


if actualSlip >= 0 %Positive slip (Acceleration control)
    if actualSlip > SlipTarget 
        setpoint = SlipTarget;
        enable = 1; % Slip Control is active
    else 
        setpoint = 0; %Can this be commented out or does it need a value
                        %when disabled
        enable = 0;
    end

elseif actualSlip < 0 %Negative slip (Braking control)
    if actualSlip < SlipTarget*-1        
        setpoint = SlipTarget*-1;
        enable = 1; 
    else
        setpoint= 0;
        enable = 0;
    end
else
    setpoint = 0;
    enable = 0;
end

== matlab function TorqueVectoring_6_1/Traction Control/RR/MATLAB Function ==
  data: enable output; actualSlip input; setpoint output; SlipTarget input
function [enable,setpoint] = slipCtrlTrigger(actualSlip,SlipTarget)


if actualSlip >= 0 %Positive slip (Acceleration control)
    if actualSlip > SlipTarget 
        setpoint = SlipTarget;
        enable = 1; % Slip Control is active
    else 
        setpoint = 0; %Can this be commented out or does it need a value
                        %when disabled
        enable = 0;
    end

elseif actualSlip < 0 %Negative slip (Braking control)
    if actualSlip < SlipTarget*-1        
        setpoint = SlipTarget*-1;
        enable = 1; 
    else
        setpoint= 0;
        enable = 0;
    end
else
    setpoint = 0;
    enable = 0;
end

== matlab function TorqueVectoring_6_1/Yaw Control/MATLAB Function ==
  data: yaw_error input; yaw_target output; Ki_yaw parameter; Kd_yaw parameter; Kp_yaw parameter; yaw_prev_error parameter
function yaw_target = fcn(yaw_error, Ki_yaw, Kd_yaw, Kp_yaw, yaw_prev_error)
dt = .001;
proportional = Kp_yaw*yaw_error;
integral = Ki_yaw*(yaw_error)*dt;
derivative = Kd_yaw*(yaw_error-yaw_prev_error)/dt;
output = proportional + integral + derivative;
yaw_prev_error = yaw_error;
yaw_target = output;

== matlab function TorqueVectoring_6_1/Torque Distribution/Torque Distribution ==
  data: Mz input; torquePer input; FLtorque output; FRtorque output; RLtorque output; RRtorque output; lambda input
function [FLtorque,FRtorque,RLtorque,RRtorque] = fcn(Mz,torquePer,lambda)
%% Torque Distribution 


%% Inputs
%FL, FR, RL, RR maxes   = maximum allowable forces at each corner
%Mz                     = Yaw moment target
%torquePer              = Torque demand as a percentage
%lambda                 = Front bias %, Lambda >.5 front biased, lambda <.5 rear biased

%If distributionStatus = 0, traction will be evenly split between all 4
%corners
distributionStatus = 1;

%% Constants
rw = .4064;
tw = 1.34;
alpha = 2*rw/tw ;                               %Constant from to wheel radius and track width; converts Mz into in forces (instead of torques)
GR = 13;                                        %Gear ratio
motorPk = 21;                                   %Peak torque output of motor                                             
tractDemand = torquePer*motorPk*GR/rw;          %Traction requested after throttle and gear train

Tf_FL=0;            %Initialization
Tf_FR=0;
Tf_RL=0;
Tf_RR=0;

momentBal=0;

%% Torque Distribution based on Peak traction tire and throttle request

if lambda <= .5 
    if Mz <= 0 % if Moment request is clockwise (Right hand turn) %Assumes weight is rear left biased
        Tf_RL = tractDemand;
        Tf_FL = tractDemand*(lambda/(1-lambda));
        if torquePer >= 0                                                           %Under Acceleration
            momentBal = Mz*(alpha) + tractDemand + tractDemand*(lambda/(1-lambda)); %moment offset
            if momentBal > 0                    %if Moment request exceed torque dme
                Tf_FR = momentBal*lambda;  
                Tf_RR = momentBal*(1-lambda);
            else
                Tf_FR = 0;
                f_RR = 0;
            end

        else                                                                            %Under Braking
            momentBal = -1*Mz*(alpha) + tractDemand + tractDemand*(lambda/(1-lambda)); %moment offset
            if momentBal < 0
                Tf_FR = momentBal*lambda;
                Tf_RR = momentBal*(1-lambda);
            else
                Tf_FR = 0;
                Tf_RR = 0;
            end
        end
    elseif Mz > 0 % if Moment request is counter clockwise (Left hand turn)
        Tf_RR = tractDemand;
        Tf_FR = tractDemand*(lambda/(1-lambda));
        if torquePer >= 0
            momentBal = -1*(Mz*alpha) + tractDemand + tractDemand*(lambda/(1-lambda)); %moment offset
            if momentBal > 0
                Tf_FL = momentBal*lambda;
                Tf_RL = momentBal*(1-lambda);
            else
                Tf_FL = 0;
                Tf_RL = 0;
            end
        else
            momentBal = 1*(Mz*alpha) + tractDemand + tractDemand*(lambda/(1-lambda));
            if momentBal < 0
                Tf_FL = momentBal*lambda;
                Tf_RL = momentBal*(1-lambda);
            else
                %Tf_FL = 0;
                %Tf_RL = 0;
            end
        end
    end

elseif lambda >.5   %Front Biased
    if Mz <= 0 % if Moment Request is clockwise (Right hand turn)
        Tf_FL = tractDemand;
        Tf_RL = tractDemand*((1-lambda)/lambda); 
        if torquePer >= 0 
            momentBal = (Mz*alpha) + tractDemand + tractDemand*((1-lambda)/lambda); %moment offset
            if momentBal > 0
                Tf_FR = momentBal*lambda;
                Tf_RR = momentBal*(1-lambda);
            else
                Tf_FR = 0;
                Tf_RR = 0;
            end
        else
            momentBal = -1*(Mz*alpha) + tractDemand + tractDemand*((1-lambda)/lambda); %moment offset
            if momentBal < 0
                Tf_FR = momentBal*lambda;
                Tf_RR = momentBal*(1-lambda);
            else
                Tf_FR = 0;
                Tf_RR = 0;
            end
        end

    elseif Mz > 0 % if Moment request is counter clockwise (Left hand turn)
        Tf_FR = tractDemand;
        Tf_RR = tractDemand*((1-lambda)/lambda); 
        if torquePer >= 0
            momentBal = -1*(Mz*alpha) + tractDemand + tractDemand*((1-lambda)/lambda); %moment offset
            if momentBal > 0
                Tf_FL = momentBal*lambda;
                Tf_RL = momentBal*(1-lambda);
            else
                Tf_FL = 0;
                Tf_RL = 0;
            end
        else
            momentBal = 1*(Mz*alpha) + tractDemand + tractDemand*((1-lambda)/lambda); %moment offset
            if momentBal < 0
                Tf_FL = momentBal*lambda;
                Tf_RL = momentBal*(1-lambda);
            else
                Tf_FL = 0;
                Tf_RL = 0;
            end
        end
    end
end

%% Assign Torques
if Tf_FL >= 0 
    if Tf_FL*rw > motorPk*GR; %Saturation Check
        FLtorque = motorPk*GR;
    else
        FLtorque = Tf_FL*rw; 
    end
else
    if Tf_FL*rw < -1*motorPk*GR %Saturation Check
        FLtorque = -1*motorPk*GR;
    else
        FLtorque = Tf_FL*rw; 
    end
end

if Tf_FR >= 0 
    if Tf_FR*rw > motorPk*GR; %Saturation Check
        FRtorque = motorPk*GR;
    else
        FRtorque = Tf_FR*rw; 
    end
else
    if Tf_FR*rw < -1*motorPk*GR %Saturation Check
        FRtorque = -1*motorPk*GR;
    else
        FRtorque = Tf_FR*rw; 
    end
end

if Tf_RL >= 0 
    if Tf_RL*rw > motorPk*GR; %Saturation Check
        RLtorque = motorPk*GR;
    else
        RLtorque = Tf_RL*rw; 
    end
else
    if Tf_RL*rw < -1*motorPk*GR %NegativeSaturation Check
        RLtorque = -1*motorPk*GR;
    else
        RLtorque = Tf_RL*rw; 
    end
end

if Tf_RR >= 0 
    if Tf_RR*rw > motorPk*GR; %Saturation Check
        RRtorque = motorPk*GR;
    else
        RRtorque = Tf_RR*rw; 
    end
else
    if Tf_RR*rw < -1*motorPk*GR %Saturation Check
        RRtorque = -1*motorPk*GR;
    else
        RRtorque = Tf_RR*rw; 
    end
end

%% Torque outputs

if distributionStatus == 0
    FLtorque = tractDemand;
    FRtorque = tractDemand;
    RLtorque = tractDemand;
    RRtorque = tractDemand;
end

== matlab function TorqueVectoring_6_1/Torque Distribution/Front-Rear Bias ==
  data: zFL input; lambda output; zFR input; zRL input; zRR input
function lambda  = FzDistribution(zFL, zFR, zRL, zRR)
                %delta removed as output

zTotal = zFL + zFR + zRL + zRR;

lambda = (zFL + zFR)/zTotal; %Front to Rear Bias %
%delta = (zFL + zRL)/zTotal; %Left to Right Bias %

== matlab function TorqueVectoring_6_1/Sine Steering Input ==
  data: u input; y output
function y = fcn(u)

A = 10;
f = .01;

y = A*sin(2*pi*f*u);

== matlab function TorqueVectoring_6_1/Torque Distribution/MATLAB Function ==
  data: u input; y output
function y = fcn(u)
if Tf_FL >= 0 
    if Tf_FL*rw > motorPk*GR; %Saturation Check
        FLtorque = motorPk*GR;
    else
        FLtorque = Tf_FL*rw; 
    end
else
    if Tf_FL*rw < -1*motorPk*GR %Saturation Check
        FLtorque = -1*motorPk*GR;
    else
        FLtorque = Tf_FL*rw; 
    end
end

if Tf_FR >= 0 
    if Tf_FR*rw > motorPk*GR; %Saturation Check
        FRtorque = motorPk*GR;
    else
        FRtorque = Tf_FR*rw; 
    end
else
    if Tf_FR*rw < -1*motorPk*GR %Saturation Check
        FRtorque = -1*motorPk*GR;
    else
        FRtorque = Tf_FR*rw; 
    end
end

if Tf_RL >= 0 
    if Tf_RL*rw > motorPk*GR; %Saturation Check
        RLtorque = motorPk*GR;
    else
        RLtorque = Tf_RL*rw; 
    end
else
    if Tf_RL*rw < -1*motorPk*GR %NegativeSaturation Check
        RLtorque = -1*motorPk*GR;
    else
        RLtorque = Tf_RL*rw; 
    end
end

if Tf_RR >= 0 
    if Tf_RR*rw > motorPk*GR; %Saturation Check
        RRtorque = motorPk*GR;
    else
        RRtorque = Tf_RR*rw; 
    end
else
    if Tf_RR*rw < -1*motorPk*GR %Saturation Check
        RRtorque = -1*motorPk*GR;
    else
        RRtorque = Tf_RR*rw; 
    end
end

== matlab function TorqueVectoring_6_1/Vehicle Dynamics Model/14 DOF MODEL/Subsys Tire/Subsys tfl/Fy Tire ==
  data: SA input; FY output; FZ input
function FY  = FYgen_H16x75LC07(SA, FZ)
%{
Coefficient values for tire are obtained through tire parser
c(1) = a0
c(2) = a1
.... etc
%}

c = [1.3662,0.0013,2.7913,7322.2407,300.0032,0.3242];
a0 = c(1);
a1 = c(2);
a2 = c(3);
a3 = c(4);
a4 = c(5);
a7 = c(6); 

C = a0;
H = 0;
E = a7;
V = 0;

D = FZ.*(a1.*FZ+a2);
BCD = a3.*sin(atan(FZ./a4).*2);
B = BCD./(C.*D);
Bx1 = B.*(SA+H);

FY = D.*sin(C.*atan(Bx1-E.*(Bx1-atan(Bx1))))+V;
end

== matlab function TorqueVectoring_6_1/Vehicle Dynamics Model/14 DOF MODEL/Subsys Tire/Subsys tfl/Fx Tire ==
  data: SL input; FZ input; FX output
function FX  = FXgen_H18x75R25B7(SL, FZ)
%Coefficient values for tire are obtained through tire parser 
%c(1) = a1...
%SL is in percentage

surface = .56; %Track surface scaling factor taken from H18x6LC07

FZ = -FZ;
c = [9.024117283527670e-04,-2.000000000004689,2.999999993293833e+03,-6.381207727102746e-04,-0.564754663496273,1.061795649571943];
b0 = c(1);
b1 = c(2);
b2 = c(3);
b3 = c(4);
b4 = c(5);
b8 = c(6);

C = b0;
H = 0;
E = b8;
V = 0;

D = FZ.*(b1.*FZ+b2);
BCD = (b3.*FZ.^2+b4.*FZ);
B = BCD./(C.*D);
Bx1 = B.*(SL+H);

FX = surface*D.*sin(C.*atan(Bx1-E.*(Bx1-atan(Bx1))))+V;
end

== matlab function TorqueVectoring_6_1/Vehicle Dynamics Model/14 DOF MODEL/Subsys Tire/Subsys tfl1/Fx Tire ==
  data: SL input; FZ input; FX output
function FX  = FXgen_H18x75R25B7(SL, FZ)
%Coefficient values for tire are obtained through tire parser 
%c(1) = a1...
%SL is in percentage

surface = .56; %Track surface scaling factor taken from H18x6LC07

FZ = -FZ;
c = [9.024117283527670e-04,-2.000000000004689,2.999999993293833e+03,-6.381207727102746e-04,-0.564754663496273,1.061795649571943];
b0 = c(1);
b1 = c(2);
b2 = c(3);
b3 = c(4);
b4 = c(5);
b8 = c(6);

C = b0;
H = 0;
E = b8;
V = 0;

D = FZ.*(b1.*FZ+b2);
BCD = (b3.*FZ.^2+b4.*FZ);
B = BCD./(C.*D);
Bx1 = B.*(SL+H);

FX = surface*D.*sin(C.*atan(Bx1-E.*(Bx1-atan(Bx1))))+V;
end

== matlab function TorqueVectoring_6_1/Vehicle Dynamics Model/14 DOF MODEL/Subsys Tire/Subsys tfl1/Fy Tire ==
  data: SA input; FY output; FZ input
function FY  = FYgen_H16x75LC07(SA, FZ)
%{
Coefficient values for tire are obtained through tire parser
c(1) = a0
c(2) = a1
.... etc
%}

c = [1.3662,0.0013,2.7913,7322.2407,300.0032,0.3242];
a0 = c(1);
a1 = c(2);
a2 = c(3);
a3 = c(4);
a4 = c(5);
a7 = c(6); 

C = a0;
H = 0;
E = a7;
V = 0;

D = FZ.*(a1.*FZ+a2);
BCD = a3.*sin(atan(FZ./a4).*2);
B = BCD./(C.*D);
Bx1 = B.*(SA+H);

FY = D.*sin(C.*atan(Bx1-E.*(Bx1-atan(Bx1))))+V;
end

== matlab function TorqueVectoring_6_1/Vehicle Dynamics Model/14 DOF MODEL/Subsys Tire/Subsys tfl2/Fx Tire ==
  data: SL input; FZ input; FX output
function FX  = FXgen_H18x75R25B7(SL, FZ)
%Coefficient values for tire are obtained through tire parser 
%c(1) = a1...
%SL is in percentage

surface = .56; %Track surface scaling factor taken from H18x6LC07

FZ = -FZ;
c = [9.024117283527670e-04,-2.000000000004689,2.999999993293833e+03,-6.381207727102746e-04,-0.564754663496273,1.061795649571943];
b0 = c(1);
b1 = c(2);
b2 = c(3);
b3 = c(4);
b4 = c(5);
b8 = c(6);

C = b0;
H = 0;
E = b8;
V = 0;

D = FZ.*(b1.*FZ+b2);
BCD = (b3.*FZ.^2+b4.*FZ);
B = BCD./(C.*D);
Bx1 = B.*(SL+H);

FX = surface*D.*sin(C.*atan(Bx1-E.*(Bx1-atan(Bx1))))+V;
end

== matlab function TorqueVectoring_6_1/Vehicle Dynamics Model/14 DOF MODEL/Subsys Tire/Subsys tfl2/Fy Tire ==
  data: SA input; FY output; FZ input
function FY  = FYgen_H16x75LC07(SA, FZ)
%{
Coefficient values for tire are obtained through tire parser
c(1) = a0
c(2) = a1
.... etc
%}

c = [1.3662,0.0013,2.7913,7322.2407,300.0032,0.3242];
a0 = c(1);
a1 = c(2);
a2 = c(3);
a3 = c(4);
a4 = c(5);
a7 = c(6); 

C = a0;
H = 0;
E = a7;
V = 0;

D = FZ.*(a1.*FZ+a2);
BCD = a3.*sin(atan(FZ./a4).*2);
B = BCD./(C.*D);
Bx1 = B.*(SA+H);

FY = D.*sin(C.*atan(Bx1-E.*(Bx1-atan(Bx1))))+V;
end

== matlab function TorqueVectoring_6_1/Vehicle Dynamics Model/14 DOF MODEL/Subsys Tire/Subsys tfl3/Fx Tire ==
  data: SL input; FZ input; FX output
function FX  = FXgen_H18x75R25B7(SL, FZ)
%Coefficient values for tire are obtained through tire parser 
%c(1) = a1...
%SL is in percentage

surface = .56; %Track surface scaling factor taken from H18x6LC07

FZ = -FZ;
c = [9.024117283527670e-04,-2.000000000004689,2.999999993293833e+03,-6.381207727102746e-04,-0.564754663496273,1.061795649571943];
b0 = c(1);
b1 = c(2);
b2 = c(3);
b3 = c(4);
b4 = c(5);
b8 = c(6);

C = b0;
H = 0;
E = b8;
V = 0;

D = FZ.*(b1.*FZ+b2);
BCD = (b3.*FZ.^2+b4.*FZ);
B = BCD./(C.*D);
Bx1 = B.*(SL+H);

FX = surface*D.*sin(C.*atan(Bx1-E.*(Bx1-atan(Bx1))))+V;
end
